simulink model "PA_Longitudinal"  (Simulink 8.7)
settings: Solver=ode8  StartTime=0.0  StopTime=300  FixedStep=0.01  RelTol=1e-3
undefined symbols (not defined in the file or in its folder): Ue, Xe
libraries: xpcutilitieslib x2, instrumentlib x2, xpcobsoletelib x2, sldrtlib x1
settings Model: Creator=Marcelo Henrique  LastModifiedBy=Marcelo  PauseTimes=150
settings DataIOCC: MaxDataPoints=10000
settings DebuggingCC: AlgebraicLoopMsg=none  StateNameClashWarn=warning

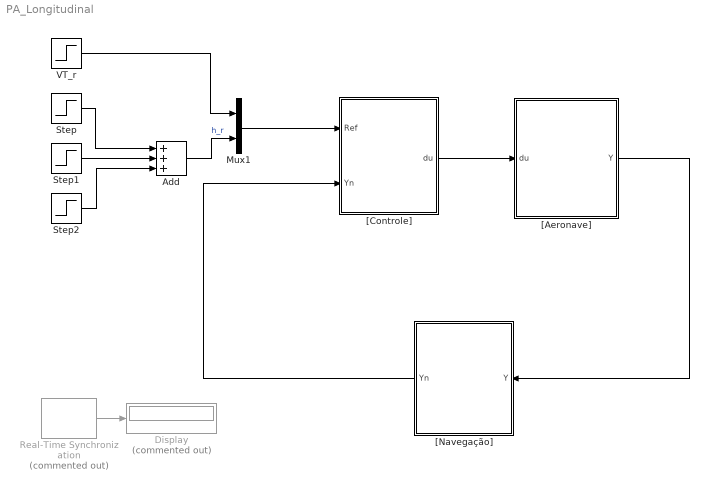
== system PA_Longitudinal ==
  Add : Sum  Inputs=+++
  Display : Display  Commented=on
  Mux1 : Mux  Inputs=2
  Real-Time Synchronization : sldrtlib/Real-Time Synchronization  Commented=on  SampleTime=0.01  MaxMissedTicks=inf  ShowMissedTicks=on  YieldWhenWaiting=on
  Step : Step  Time=50  Before=-Xe(12)  After=-Xe(12)+25  SampleTime=0
  Step1 : Step  Time=150  After=-50  SampleTime=0
  Step2 : Step  Time=250  After=25  SampleTime=0
  VT_r : Step  Time=0  Before=norm(Xe(1:3))  After=norm(Xe(1:3))  SampleTime=0
  "[Aeronave]" : Subsystem
  "[Controle]" : Subsystem
  "[Navegação]" : Subsystem
  wires:
  "[Navegação]"/1(Yn) -> "[Controle]"/2(Yn)
  "[Controle]"/1(du) -> "[Aeronave]"/1(du)
  "[Aeronave]"/1(Y) -> "[Navegação]"/1(Y)
  VT_r/1 -> Mux1/1
  Add/1 -> Mux1/2  "h_r"
  Step/1 -> Add/1
  Step1/1 -> Add/2
  Step2/1 -> Add/3
  Mux1/1 -> "[Controle]"/1(Ref)
  Real-Time Synchronization/1 -> Display/1

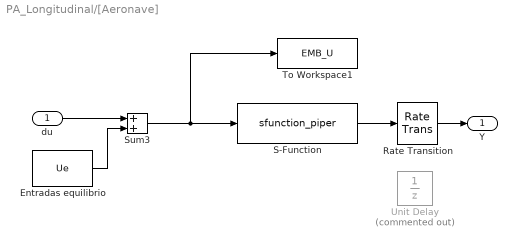
== system PA_Longitudinal/[Aeronave] ==
  du : Inport
  Entradas equilibrio : Constant  Value=Ue
  Rate Transition : RateTransition  OutPortSampleTime=0.01
  S-Function : S-Function  FunctionName=sfunction_piper  Parameters=par_gen,par_aero,par_prop, Xe  SFunctionDeploymentMode=off  EnableBusSupport=off
  Sum3 : Sum
  To Workspace1 : ToWorkspace  VariableName=EMB_U  SaveFormat=Timeseries  SampleTime=-1
  Unit Delay : UnitDelay  Commented=on  SampleTime=-1
  Y : Outport
  wires:
  S-Function/1 -> Rate Transition/1
  du/1 -> Sum3/1
  Entradas equilibrio/1 -> Sum3/2
  Sum3/1 -> S-Function/1, To Workspace1/1
  Rate Transition/1 -> Y/1

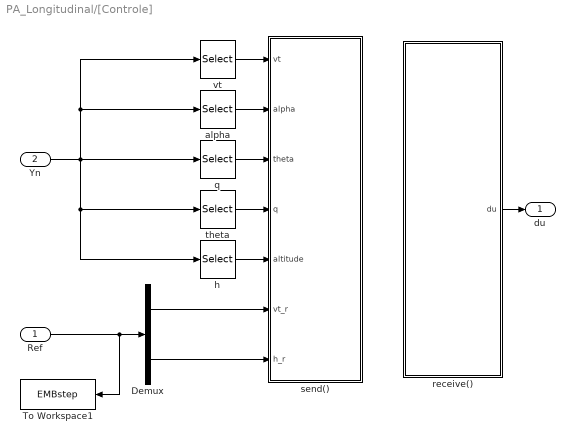
== system PA_Longitudinal/[Controle] ==
  Ref : Inport
  Yn : Inport  Port=2
  Demux : Demux  Outputs=2
  To Workspace1 : ToWorkspace  VariableName=EMBstep  SaveFormat=Timeseries  SampleTime=-1
  alpha : Selector  InputPortWidth=5  IndexOptions=Index vector (dialog)  Indices=[2]  OutputSizes=1
  h : Selector  InputPortWidth=5  IndexOptions=Index vector (dialog)  Indices=[5]  OutputSizes=1
  q : Selector  InputPortWidth=5  IndexOptions=Index vector (dialog)  Indices=[3]  OutputSizes=1
  receive() : Subsystem
  send() : Subsystem
  theta : Selector  InputPortWidth=5  IndexOptions=Index vector (dialog)  Indices=[4]  OutputSizes=1
  vt : Selector  InputPortWidth=5  IndexOptions=Index vector (dialog)  Indices=[1]  OutputSizes=1
  du : Outport
  wires:
  receive()/1(du) -> du/1
  vt/1 -> send()/1(vt)
  alpha/1 -> send()/2(alpha)
  q/1 -> send()/3(theta)
  theta/1 -> send()/4(q)
  h/1 -> send()/5(altitude)
  Yn/1 -> h/1, theta/1, alpha/1, vt/1, q/1
  Ref/1 -> To Workspace1/1, Demux/1
  Demux/1 -> send()/6(vt_r)
  Demux/2 -> send()/7(h_r)

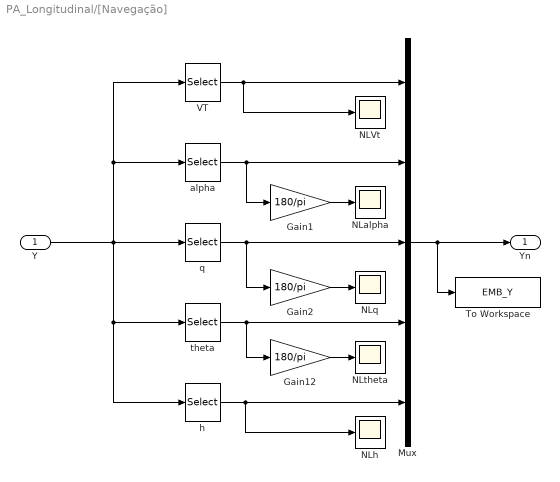
== system PA_Longitudinal/[Navegação] ==
  Y : Inport
  Gain1 : Gain  Gain=180/pi
  Gain12 : Gain  Gain=180/pi
  Gain2 : Gain  Gain=180/pi
  Mux : Mux  Inputs=5
  NLVt : Scope
  NLalpha : Scope
  NLh : Scope
  NLq : Scope
  NLtheta : Scope
  To Workspace : ToWorkspace  VariableName=EMB_Y  SaveFormat=Timeseries  SampleTime=-1
  VT : Selector  InputPortWidth=12  IndexOptions=Index vector (dialog)  Indices=[1]  OutputSizes=1
  alpha : Selector  InputPortWidth=12  IndexOptions=Index vector (dialog)  Indices=[2]  OutputSizes=1
  h : Selector  InputPortWidth=12  IndexOptions=Index vector (dialog)  Indices=[12]  OutputSizes=1
  q : Selector  InputPortWidth=12  IndexOptions=Index vector (dialog)  Indices=[5]  OutputSizes=1
  theta : Selector  InputPortWidth=12  IndexOptions=Index vector (dialog)  Indices=[8]  OutputSizes=1
  Yn : Outport
  wires:
  Y/1 -> h/1, theta/1, VT/1, alpha/1, q/1
  Gain12/1 -> NLtheta/1
  VT/1 -> NLVt/1, Mux/1
  theta/1 -> Gain12/1, Mux/4
  h/1 -> NLh/1, Mux/5
  Gain1/1 -> NLalpha/1
  alpha/1 -> Gain1/1, Mux/2
  Gain2/1 -> NLq/1
  q/1 -> Gain2/1, Mux/3
  Mux/1 -> To Workspace/1, Yn/1

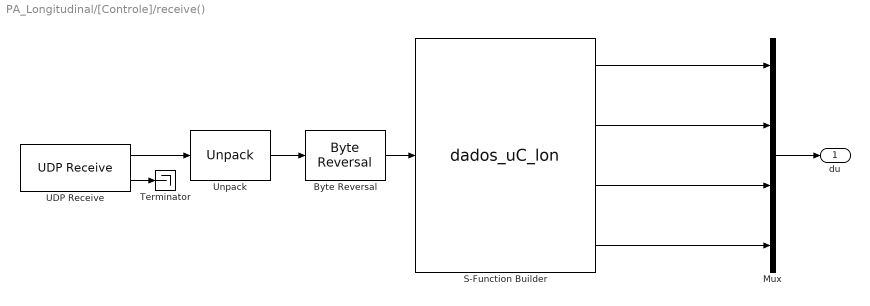
== system PA_Longitudinal/[Controle]/receive() ==
  Byte Reversal : xpcutilitieslib/Byte Reversal   numInp=1
  Mux : Mux
  S-Function Builder : S-Function  InitFcn=try, set_param(gcb,'FunctionName','dados_uC_lon'), end  FunctionName=dados_uC_lon  SFunctionModules=dados_uC_lon_wrapper  WizardData=DataTag0  SFunctionDeploymentMode=off  EnableBusSupport=off  mask(S-Function Builder){}
      mask help: Simulink:masks:SFunctionBuilder_MD
      mask init:
      | val = [[.9  0.75 0.75 1 1 .9 .9 1]',[1 1 0.75 0.75 .9 .9 1 .9]'];try , sys = get_param(gcb,'SfunBuilderFcnName');if isempty(sys), sys = get_param(gcb,'FunctionName'); end,catch, sys = get_param(gcb,'FunctionName'); end
      settings: CopyFcn=set_param(gcbh,'LinkStatus','none')  PreSaveFcn=try, set_param(gcb,'FunctionName','dados_uC_lon'), end  OpenFcn=sfunctionwizard(gcbh)
      mask Display: plot(val(:,1),val(:,2)),disp(sys), port_label('input',1,'control'), port_label('output',1,'ut'), port_label('output',2,'ue'), port_label('output',3,'ua'), port_label('output',4,'ur')
  Terminator : Terminator
  UDP Receive : instrumentlib/UDP Receive  Host=192.168.1.101  Port=45004  LocalPort=45000  DataSize=16  EnableBlockingMode=off  Timeout=10  SampleTime=0.01  DataType=uint8  ByteOrder=BigEndian
  Unpack : xpcobsoletelib/Utilities/Unpack   dimensions={[1 16]}  datatypes={'uint8'}  byteAlign=1
  du : Outport
  wires:
  UDP Receive/1 -> Unpack/1
  Unpack/1 -> Byte Reversal/1
  Byte Reversal/1 -> S-Function Builder/1
  UDP Receive/2 -> Terminator/1
  S-Function Builder/3 -> Mux/3
  S-Function Builder/4 -> Mux/4
  Mux/1 -> du/1
  S-Function Builder/2 -> Mux/2
  S-Function Builder/1 -> Mux/1

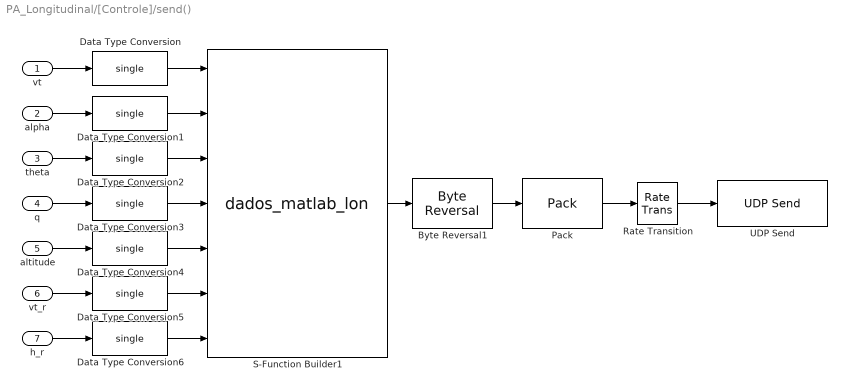
== system PA_Longitudinal/[Controle]/send() ==
  vt : Inport
  alpha : Inport  Port=2
  theta : Inport  Port=3
  q : Inport  Port=4
  altitude : Inport  Port=5
  vt_r : Inport  Port=6
  h_r : Inport  Port=7
  Byte Reversal1 : xpcutilitieslib/Byte Reversal   numInp=1
  Data Type Conversion{,1..6} (7 alike) : DataTypeConversion  OutDataTypeStr=single
  Pack : xpcobsoletelib/Utilities/Pack   datatypes={'uint8'}  byteAlign=1
  Rate Transition : RateTransition  OutPortSampleTime=0.01
  S-Function Builder1 : S-Function  InitFcn=try, set_param(gcb,'FunctionName','dados_matlab_lon'), end  FunctionName=dados_matlab_lon  SFunctionModules=dados_matlab_lon_wrapper  WizardData=DataTag1  SFunctionDeploymentMode=off  EnableBusSupport=off  mask(S-Function Builder){}
      mask help: Simulink:masks:SFunctionBuilder_MD
      mask init: same as PA_Longitudinal/[Controle]/receive()/S-Function Builder
      settings: CopyFcn=set_param(gcbh,'LinkStatus','none')  PreSaveFcn=try, set_param(gcb,'FunctionName','dados_matlab_lon'), end  OpenFcn=sfunctionwizard(gcbh)
      mask Display: plot(val(:,1),val(:,2)),disp(sys), port_label('input',1,'vt'), port_label('input',2,'alpha'), port_label('input',3,'q'), port_label('input',4,'theta'), port_label('input',5,'altitude'), port_label('input',6,'vt_r'), port_label('input',7,'h_r'), port_label('output',1,'data')
  UDP Send : instrumentlib/UDP Send  Host=192.168.1.101  Port=45004  LocalPort=45001  EnableBlockingMode=on  ByteOrder=BigEndian
  wires:
  Byte Reversal1/1 -> Pack/1
  vt/1 -> Data Type Conversion/1
  S-Function Builder1/1 -> Byte Reversal1/1
  alpha/1 -> Data Type Conversion1/1
  theta/1 -> Data Type Conversion2/1
  q/1 -> Data Type Conversion3/1
  altitude/1 -> Data Type Conversion4/1
  Data Type Conversion/1 -> S-Function Builder1/1
  Data Type Conversion1/1 -> S-Function Builder1/2
  Data Type Conversion2/1 -> S-Function Builder1/3
  vt_r/1 -> Data Type Conversion5/1
  Data Type Conversion5/1 -> S-Function Builder1/6
  Data Type Conversion4/1 -> S-Function Builder1/5
  Data Type Conversion3/1 -> S-Function Builder1/4
  Pack/1 -> Rate Transition/1
  Rate Transition/1 -> UDP Send/1
  Data Type Conversion6/1 -> S-Function Builder1/7
  h_r/1 -> Data Type Conversion6/1
